simulink model "SMCtest"  (R2023b)
settings: Solver=FixedStepAuto  StartTime=0.0  StopTime=50  FixedStep=0.0001  RelTol=1e-3
InitFcn:
  | %% 反步法与自适应参数
  | % % k = 10;
  | % m = 10;
  | %
  | % k1 = 25;
  | % k2 = 25;
  | %% 滑模参数
  | c = 30;
  | p = 30;
  | theta = 20;
  | 
  | m = 10;
undefined symbols (not defined in the file or in its folder): k1, k2
settings Model: Creator=崔晓凯  LastModifiedBy=Hitsz
settings DebuggingCC: UnconnectedInputMsg=warning  UnconnectedOutputMsg=warning  UnconnectedLineMsg=warning
settings ModelReferenceCC: EnableRefExpFcnMdlSchedulingChecks=on
settings RTWCC: DLArmComputeVersion=19.05

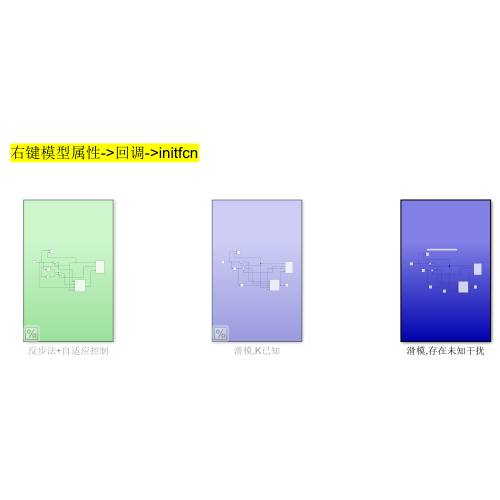
[thumbnail: Simulink's stored preview of the top-level diagram]
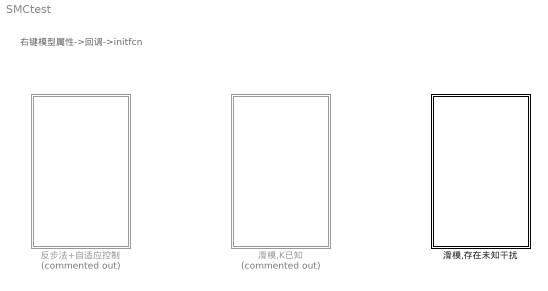
== system SMCtest ==
  note: 右键模型属性->回调->initfcn
  反步法+自适应控制 : Subsystem  Commented=on
  滑模,K已知 : Subsystem  Commented=on
  滑模,存在未知干扰 : Subsystem

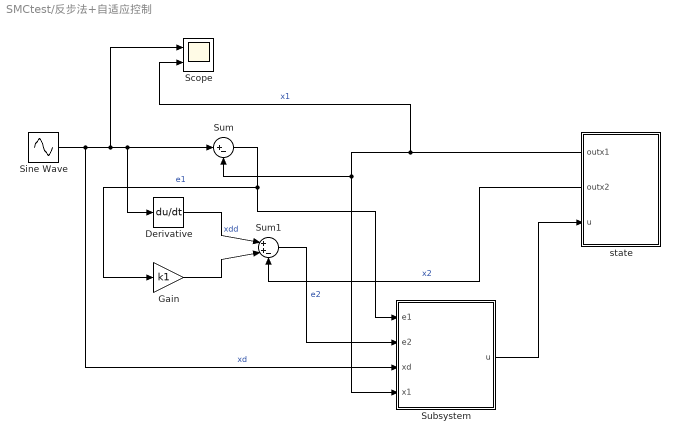
== system SMCtest/反步法+自适应控制 ==
  Derivative : Derivative
  Gain : Gain  Gain=k1
  Scope : Scope  NumInputPorts=2
  Sine Wave : Sin  Bias=5  SampleTime=0
  Subsystem : Subsystem
  Sum : Sum  Inputs=|+-
  Sum1 : Sum  Inputs=|++-
  state : Subsystem
      settings: PortSchema="{\"entries\":[{\"content\":{\"sides\":[{\"content\":{\"connectorIds\":[\"Out1\",\"Out2\",\"In1\"]},\"type\":\"ConnectorPlacement.EquallySpacedRectSide\",\"uuid\":\"d6ff9530-3cd8-44b3-9e02-2ac40466835c\"},{\"content\":{\"connectorIds\":[],\"side\":\"RIGHT\"},\"type\":\"ConnectorPlacement.EquallySpacedRectSide\",\"uuid\":\"a7c79afe-87fc-43ce-be47-0aa427f252c3\"},{\"content\":{\"connectorIds\":[],\"side\":\"TOP\"},\"type\":\"ConnectorPlacement.EquallySpacedRectSide\",\"uuid\":\"01a8c9c6-0152-4abd-adba-4721d7ab5cc8\"}]},\"type\":\"ConnectorPlacement.EquallySpacedConnector\",\"uuid\":\"4c659116-fed0-430d-b09c-79e2d5ab99b5\"}],\"packageUris\":[\"http://schema.mathworks.com/mf0/Connector/R2020b\"],\"version\":\"1.0\"}"
  wires:
  Derivative/1 -> Sum1/1  "xdd"
  state/2(outx2) -> Sum1/3  "x2"
  Sine Wave/1 -> Subsystem/3(xd), Scope/1, Sum/1, Derivative/1  "xd"
  Sum/1 -> Subsystem/1(e1), Gain/1  "e1"
  Subsystem/1(u) -> state/1(u)
  state/1(outx1) -> Scope/2, Subsystem/4(x1), Sum/2  "x1"
  Gain/1 -> Sum1/2
  Sum1/1 -> Subsystem/2(e2)  "e2"

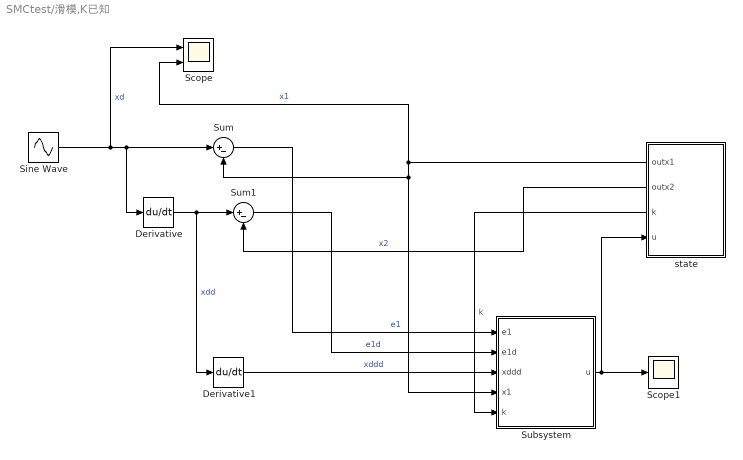
== system SMCtest/滑模,K已知 ==
  Derivative : Derivative
  Derivative1 : Derivative
  Scope : Scope  NumInputPorts=2
  Scope1 : Scope
  Sine Wave : Sin  Amplitude=5  Frequency=0.5  SampleTime=0
  Subsystem : Subsystem
  Sum : Sum  Inputs=|+-
  Sum1 : Sum  Inputs=|+-
  state : Subsystem
      settings: PortSchema="{\"entries\":[{\"content\":{\"sides\":[{\"content\":{\"connectorIds\":[\"Out1\",\"Out2\",\"Out3\",\"In1\"]},\"type\":\"ConnectorPlacement.EquallySpacedRectSide\",\"uuid\":\"d6ff9530-3cd8-44b3-9e02-2ac40466835c\"},{\"content\":{\"side\":\"RIGHT\"},\"type\":\"ConnectorPlacement.EquallySpacedRectSide\",\"uuid\":\"a7c79afe-87fc-43ce-be47-0aa427f252c3\"},{\"content\":{\"side\":\"TOP\"},\"type\":\"ConnectorPlacement.EquallySpacedRectSide\",\"uuid\":\"01a8c9c6-0152-4abd-adba-4721d7ab5cc8\"}]},\"type\":\"ConnectorPlacement.EquallySpacedConnector\",\"uuid\":\"4c659116-fed0-430d-b09c-79e2d5ab99b5\"}],\"packageUris\":[\"http://schema.mathworks.com/mf0/Connector/R2020b\"],\"version\":\"1.0\"}"
  wires:
  Sine Wave/1 -> Derivative/1, Sum/1, Scope/1  "xd"
  state/1(outx1) -> Scope/2, Subsystem/4(x1), Sum/2  "x1"
  state/2(outx2) -> Sum1/2  "x2"
  Sum1/1 -> Subsystem/2(e1d)  "e1d"
  Sum/1 -> Subsystem/1(e1)  "e1"
  Subsystem/1(u) -> Scope1/1, state/1(u)
  Derivative/1 -> Derivative1/1, Sum1/1  "xdd"
  Derivative1/1 -> Subsystem/3(xddd)  "xddd"
  state/3(k) -> Subsystem/5(k)  "k"

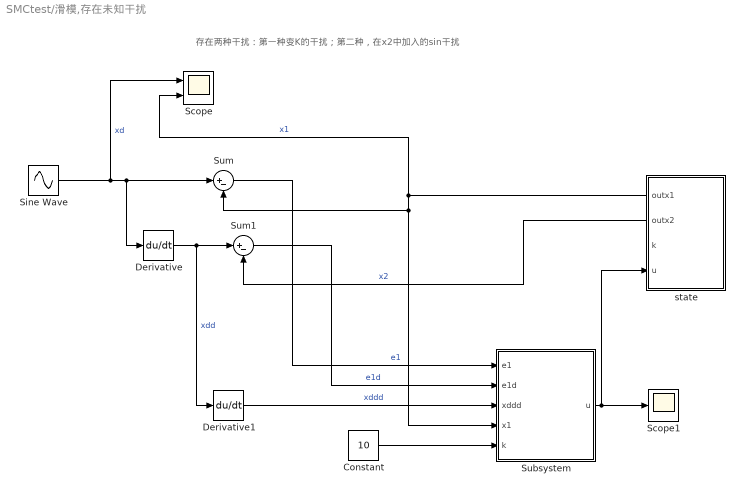
== system SMCtest/滑模,存在未知干扰 ==
  note: 存在两种干扰：第一种变K的干扰；第二种，在x2中加入的sin干扰
  Constant : Constant  Value=10
  Derivative : Derivative
  Derivative1 : Derivative
  Scope : Scope  NumInputPorts=2
  Scope1 : Scope
  Sine Wave : Sin  Amplitude=5  Frequency=0.5  SampleTime=0
  Subsystem : Subsystem
  Sum : Sum  Inputs=|+-
  Sum1 : Sum  Inputs=|+-
  state : Subsystem
      settings: PortSchema="{\"entries\":[{\"content\":{\"sides\":[{\"content\":{\"connectorIds\":[\"Out1\",\"Out2\",\"Out3\",\"In1\"]},\"type\":\"ConnectorPlacement.EquallySpacedRectSide\",\"uuid\":\"d6ff9530-3cd8-44b3-9e02-2ac40466835c\"},{\"content\":{\"side\":\"RIGHT\"},\"type\":\"ConnectorPlacement.EquallySpacedRectSide\",\"uuid\":\"a7c79afe-87fc-43ce-be47-0aa427f252c3\"},{\"content\":{\"side\":\"TOP\"},\"type\":\"ConnectorPlacement.EquallySpacedRectSide\",\"uuid\":\"01a8c9c6-0152-4abd-adba-4721d7ab5cc8\"}]},\"type\":\"ConnectorPlacement.EquallySpacedConnector\",\"uuid\":\"4c659116-fed0-430d-b09c-79e2d5ab99b5\"}],\"packageUris\":[\"http://schema.mathworks.com/mf0/Connector/R2020b\"],\"version\":\"1.0\"}"
  wires:
  Sine Wave/1 -> Derivative/1, Sum/1, Scope/1  "xd"
  state/1(outx1) -> Scope/2, Subsystem/4(x1), Sum/2  "x1"
  state/2(outx2) -> Sum1/2  "x2"
  Sum1/1 -> Subsystem/2(e1d)  "e1d"
  Sum/1 -> Subsystem/1(e1)  "e1"
  Subsystem/1(u) -> Scope1/1, state/1(u)
  Derivative/1 -> Derivative1/1, Sum1/1  "xdd"
  Derivative1/1 -> Subsystem/3(xddd)  "xddd"
  Constant/1 -> Subsystem/5(k)

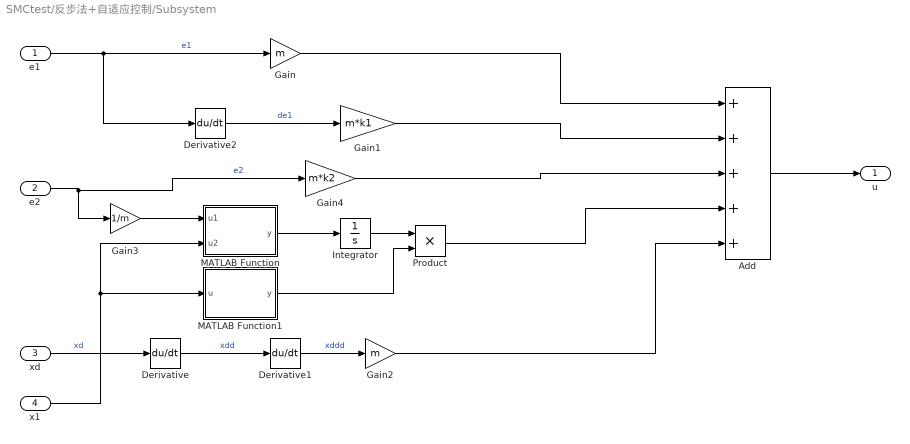
== system SMCtest/反步法+自适应控制/Subsystem ==
  e1 : Inport
  e2 : Inport  Port=2
  xd : Inport  Port=3
  x1 : Inport  Port=4
  Add : Sum  Inputs=+++++
  Derivative : Derivative
  Derivative1 : Derivative
  Derivative2 : Derivative
  Gain : Gain  Gain=m
  Gain1 : Gain  Gain=m*k1
  Gain2 : Gain  Gain=m
  Gain3 : Gain  Gain=1/m
  Gain4 : Gain  Gain=m*k2
  Integrator : Integrator
  MATLAB Function : MATLAB Function  TreatAsAtomicUnit=on
  MATLAB Function1 : MATLAB Function  TreatAsAtomicUnit=on
  Product : Product
  u : Outport
  wires:
  e1/1 -> Derivative2/1, Gain/1  "e1"
  xd/1 -> Derivative/1  "xd"
  Derivative/1 -> Derivative1/1  "xdd"
  Derivative1/1 -> Gain2/1  "xddd"
  Gain/1 -> Add/1
  Derivative2/1 -> Gain1/1  "de1"
  Gain1/1 -> Add/2
  Gain2/1 -> Add/5
  e2/1 -> Gain4/1, Gain3/1  "e2"
  Gain3/1 -> MATLAB Function/1(u1)
  x1/1 -> MATLAB Function/2(u2), MATLAB Function1/1(u)
  MATLAB Function/1(y) -> Integrator/1
  Integrator/1 -> Product/1
  Product/1 -> Add/4
  MATLAB Function1/1(y) -> Product/2
  Gain4/1 -> Add/3
  Add/1 -> u/1

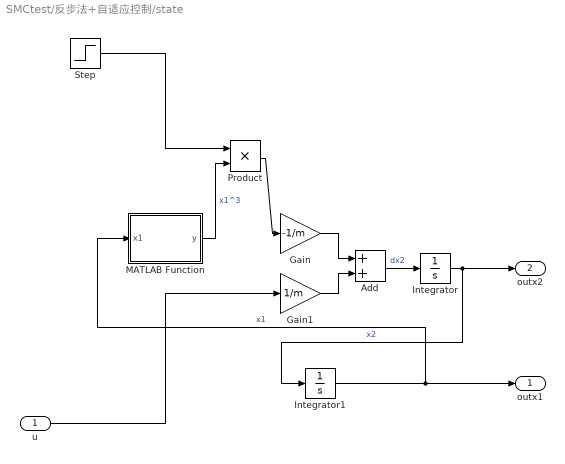
== system SMCtest/反步法+自适应控制/state ==
  u : Inport
  Add : Sum
  Gain : Gain  Gain=-1/m
  Gain1 : Gain  Gain=1/m
  Integrator : Integrator
  Integrator1 : Integrator
  MATLAB Function : MATLAB Function  TreatAsAtomicUnit=on
  Product : Product
  Step : Step  Time=5  Before=10  After=5  SampleTime=0
  outx1 : Outport
  outx2 : Outport  Port=2
  wires:
  u/1 -> Gain1/1
  Gain/1 -> Add/1
  Gain1/1 -> Add/2
  Add/1 -> Integrator/1  "dx2"
  Integrator/1 -> Integrator1/1, outx2/1  "x2"
  Integrator1/1 -> MATLAB Function/1(x1), outx1/1  "x1"
  Step/1 -> Product/1
  MATLAB Function/1(y) -> Product/2  "x1^3"
  Product/1 -> Gain/1

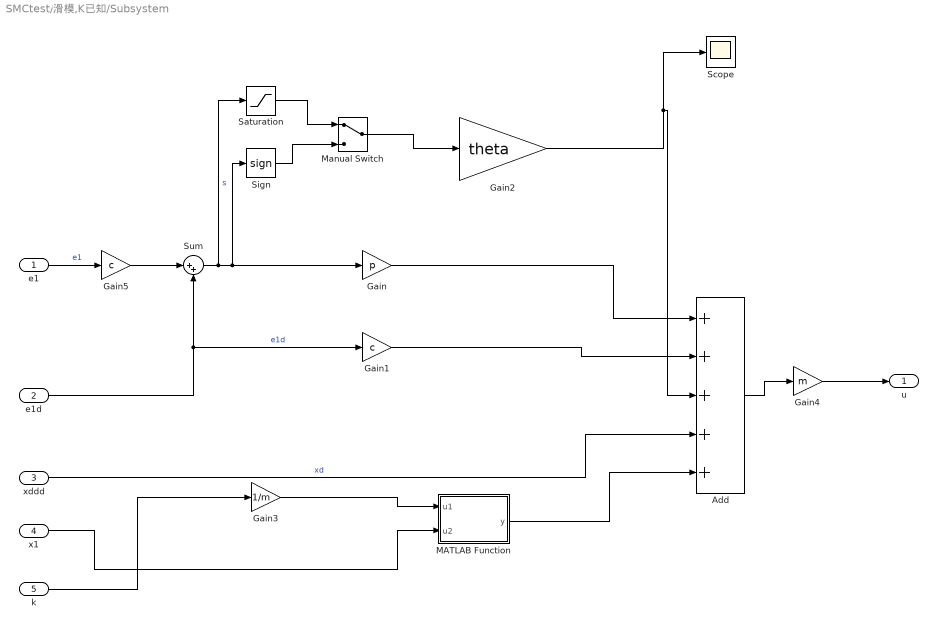
== system SMCtest/滑模,K已知/Subsystem ==
  e1 : Inport
  e1d : Inport  Port=2
  xddd : Inport  Port=3
  x1 : Inport  Port=4
  k : Inport  Port=5
  Add : Sum  Inputs=+++++
  Gain : Gain  Gain=p
  Gain1 : Gain  Gain=c
  Gain2 : Gain  Gain=theta
  Gain3 : Gain  Gain=1/m
  Gain4 : Gain  Gain=m
  Gain5 : Gain  Gain=c
  MATLAB Function : MATLAB Function  TreatAsAtomicUnit=on
  Manual Switch : ManualSwitch
  Saturation : Saturate
  Scope : Scope
  Sign : Signum
  Sum : Sum  Inputs=|++
  u : Outport
  wires:
  Add/1 -> Gain4/1
  Gain3/1 -> MATLAB Function/1(u1)
  e1/1 -> Gain5/1  "e1"
  Gain5/1 -> Sum/1
  e1d/1 -> Gain1/1, Sum/2  "e1d"
  Sum/1 -> Saturation/1, Sign/1, Gain/1  "s"
  k/1 -> Gain3/1
  x1/1 -> MATLAB Function/2(u2)
  MATLAB Function/1(y) -> Add/5
  Gain/1 -> Add/1
  Gain1/1 -> Add/2
  xddd/1 -> Add/4  "xd"
  Gain4/1 -> u/1
  Gain2/1 -> Scope/1, Add/3
  Saturation/1 -> Manual Switch/1
  Sign/1 -> Manual Switch/2
  Manual Switch/1 -> Gain2/1

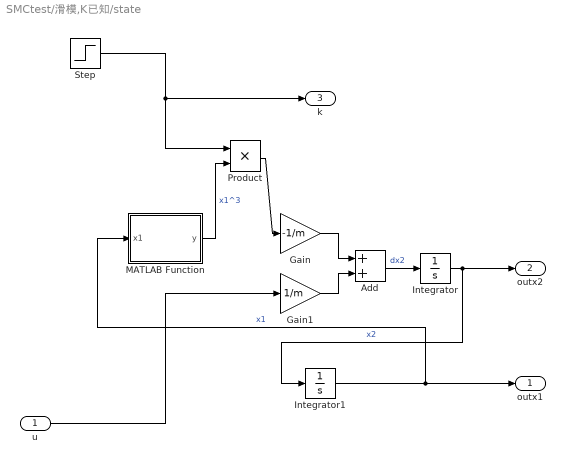
== system SMCtest/滑模,K已知/state ==
  u : Inport
  Add : Sum
  Gain : Gain  Gain=-1/m
  Gain1 : Gain  Gain=1/m
  Integrator : Integrator
  Integrator1 : Integrator
  MATLAB Function : MATLAB Function  TreatAsAtomicUnit=on
  Product : Product
  Step : Step  Time=5  Before=10  After=100  SampleTime=0
  outx1 : Outport
  outx2 : Outport  Port=2
  k : Outport  Port=3
  wires:
  Product/1 -> Gain/1
  MATLAB Function/1(y) -> Product/2  "x1^3"
  Step/1 -> Product/1, k/1
  Integrator1/1 -> outx1/1, MATLAB Function/1(x1)  "x1"
  Integrator/1 -> outx2/1, Integrator1/1  "x2"
  Add/1 -> Integrator/1  "dx2"
  Gain1/1 -> Add/2
  Gain/1 -> Add/1
  u/1 -> Gain1/1

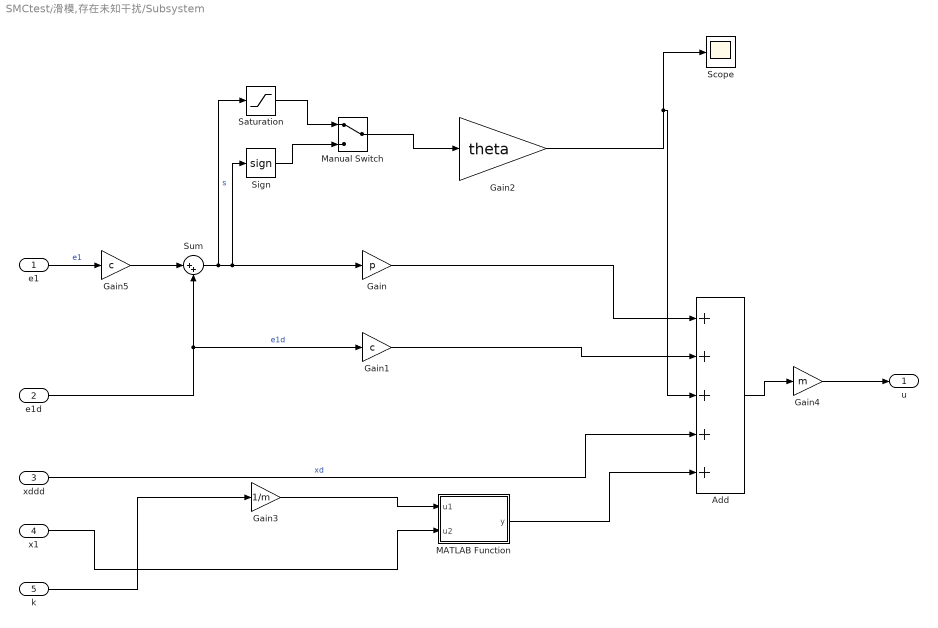
== system SMCtest/滑模,存在未知干扰/Subsystem ==
  e1 : Inport
  e1d : Inport  Port=2
  xddd : Inport  Port=3
  x1 : Inport  Port=4
  k : Inport  Port=5
  Add : Sum  Inputs=+++++
  Gain : Gain  Gain=p
  Gain1 : Gain  Gain=c
  Gain2 : Gain  Gain=theta
  Gain3 : Gain  Gain=1/m
  Gain4 : Gain  Gain=m
  Gain5 : Gain  Gain=c
  MATLAB Function : MATLAB Function  TreatAsAtomicUnit=on
  Manual Switch : ManualSwitch
  Saturation : Saturate
  Scope : Scope
  Sign : Signum
  Sum : Sum  Inputs=|++
  u : Outport
  wires:
  Add/1 -> Gain4/1
  Gain3/1 -> MATLAB Function/1(u1)
  e1/1 -> Gain5/1  "e1"
  Gain5/1 -> Sum/1
  e1d/1 -> Gain1/1, Sum/2  "e1d"
  Sum/1 -> Saturation/1, Sign/1, Gain/1  "s"
  k/1 -> Gain3/1
  x1/1 -> MATLAB Function/2(u2)
  MATLAB Function/1(y) -> Add/5
  Gain/1 -> Add/1
  Gain1/1 -> Add/2
  xddd/1 -> Add/4  "xd"
  Gain4/1 -> u/1
  Gain2/1 -> Scope/1, Add/3
  Saturation/1 -> Manual Switch/1
  Sign/1 -> Manual Switch/2
  Manual Switch/1 -> Gain2/1

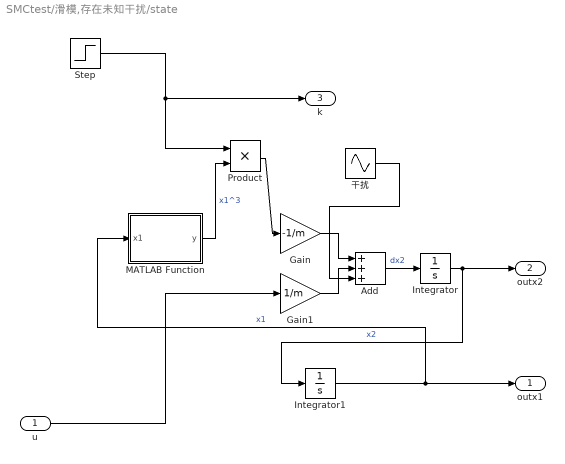
== system SMCtest/滑模,存在未知干扰/state ==
  u : Inport
  Add : Sum  Inputs=+++
  Gain : Gain  Gain=-1/m
  Gain1 : Gain  Gain=1/m
  Integrator : Integrator
  Integrator1 : Integrator
  MATLAB Function : MATLAB Function  TreatAsAtomicUnit=on
  Product : Product
  Step : Step  Time=25  Before=10  After=100  SampleTime=0
  干扰 : Sin  Amplitude=10  Frequency=2  Phase=pi/2  SampleTime=0
  outx1 : Outport
  outx2 : Outport  Port=2
  k : Outport  Port=3
  wires:
  Product/1 -> Gain/1
  MATLAB Function/1(y) -> Product/2  "x1^3"
  Step/1 -> Product/1, k/1
  Integrator1/1 -> outx1/1, MATLAB Function/1(x1)  "x1"
  Integrator/1 -> outx2/1, Integrator1/1  "x2"
  Add/1 -> Integrator/1  "dx2"
  Gain1/1 -> Add/2
  Gain/1 -> Add/1
  u/1 -> Gain1/1
  干扰/1 -> Add/3

== matlab function SMCtest/反步法+自适应控制/state/MATLAB Function ==
  data: x1 input; y output
function y = fcn(x1)

y = x1^3;

== matlab function SMCtest/反步法+自适应控制/Subsystem/MATLAB Function1 ==
  data: u input; y output
function y = fcn(u)

y = u^3;

== matlab function SMCtest/滑模,K已知/Subsystem/MATLAB Function ==
  data: u1 input; y output; u2 input
function y = fcn(u1,u2)

y = u1*u2^3;

== matlab function SMCtest/滑模,存在未知干扰/Subsystem/MATLAB Function ==
  data: u1 input; y output; u2 input
function y = fcn(u1,u2)

y = u1*u2^3;

== matlab function SMCtest/滑模,K已知/state/MATLAB Function ==
  data: x1 input; y output
function y = fcn(x1)

y = x1^3;

== matlab function SMCtest/滑模,存在未知干扰/state/MATLAB Function ==
  data: x1 input; y output
function y = fcn(x1)

y = x1^3;

== matlab function SMCtest/反步法+自适应控制/Subsystem/MATLAB Function ==
  data: u1 input; y output; u2 input
function y = fcn(u1,u2)

y = u1*u2^3;
